simulink model "baseline_auto_parcel_loading_process"  (R2026a)
settings: Solver=VariableStepAuto  StopTime=500  MaxStep=0.05
libraries: sim3dlib x36
(part 3 of 5)

== matlab function baseline_auto_parcel_loading_process/Sim3DMappingFunction ==
  data: platform_z input; platform_x output; rotator_angle input; pusher_pos input; stopper_pos input; platform_fold_angle input; platform_y output; platform_z_3d output; platform_translation output; platform_rotation output; platform_scale output; rotator_x output; rotator_y output; rotator_z output; rotator_yaw output; rotator_translation output; rotator_rotation output; rotator_scale output; pusher_x output; pusher_y output; pusher_z output; pusher_translation output; pusher_rotation output; pusher_scale output; stopper1_translation output; stopper2_translation output; stopper3_translation output; stopper_rotation output; stopper_scale output; mission_phase input
function [platform_x, platform_y, platform_z_3d, platform_translation, platform_rotation, platform_scale, ...
    rotator_x, rotator_y, rotator_z, rotator_yaw, rotator_translation, rotator_rotation, rotator_scale, ...
    pusher_x, pusher_y, pusher_z, pusher_translation, pusher_rotation, pusher_scale, ...
    stopper1_translation, stopper2_translation, stopper3_translation, stopper_rotation, stopper_scale] = ...
    Sim3DMappingFunction(platform_z, rotator_angle, pusher_pos, stopper_pos, platform_fold_angle, mission_phase)
% Sim3DMappingFunction
% Simulink 제어 신호를 3D 객체 위치/회전 신호로 변환한다.
%
% 입력:
% platform_z          : 실제 플랫폼 높이
% rotator_angle       : 플랫폼 위 회전판 yaw 각도
% pusher_pos          : 푸셔 전진 위치
% stopper_pos         : 스토퍼 위치, 1=세움, 0=접힘
% platform_fold_angle : 플랫폼 접힘 각도, 0=펼침, pi/2=접힘
% mission_phase       : 0=상차, 1=하차 준비/하차, 2=미션 완료

% =========================
% 기준 위치
% =========================
platform_base_x = 0.0;
platform_base_y = -0.35;

rotator_offset_x = 0.0;
rotator_offset_y = 0.0;
rotator_offset_z = 0.02;

pusher_offset_y_home = -0.16;
pusher_offset_z = 0.055;

% =========================
% 층 높이
% =========================
z_floor1 = 0.00;
z_floor2 = 0.27;
z_floor3 = 0.54;

% =========================
% 플랫폼 위치
% =========================
platform_x = platform_base_x;
platform_y = platform_base_y;
platform_z_visual_offset = -0.02;
platform_z_3d = platform_z + platform_z_visual_offset;

platform_translation = [platform_x, platform_y, platform_z_3d];

% platform_fold_angle:
% 0      = 펼침
% pi/2   = 접힘
%
% 접히는 축이 이상하면 여기만 바꾸면 됨.
platform_rotation = [platform_fold_angle, 0, 0];

platform_scale = [1, 1, 1];

% 거의 펼쳐진 상태인지 판단
platform_deployed = 0;
if platform_fold_angle < 0.05
    platform_deployed = 1;
end

% =========================
% 회전판 위치/회전
% =========================
rotator_x = platform_x + rotator_offset_x;
rotator_y = platform_y + rotator_offset_y;
rotator_z = platform_z_3d + rotator_offset_z;
rotator_yaw = rotator_angle;

if platform_deployed > 0.5
    rotator_translation = [rotator_x, rotator_y, rotator_z];
    rotator_rotation    = [0, 0, rotator_yaw];
    rotator_scale       = [1, 1, 1];
else
    % 플랫폼이 접힌 상태에서는 회전판 숨김
    rotator_translation = [rotator_x, rotator_y, -10.0];
    rotator_rotation    = [0, 0, 0];
    rotator_scale       = [1, 1, 1];
end

% =========================
% 푸셔 위치
% =========================
pusher_x = platform_x;
pusher_y = platform_y + pusher_offset_y_home + pusher_pos;
pusher_z = platform_z_3d + pusher_offset_z;

if platform_deployed > 0.5
    pusher_translation = [pusher_x, pusher_y, pusher_z];
    pusher_rotation    = [0, 0, 0];
    pusher_scale       = [1, 1, 1];
else
    % 플랫폼이 접힌 상태에서는 푸셔 숨김
    pusher_translation = [pusher_x, pusher_y, -10.0];
    pusher_rotation    = [0, 0, 0];
    pusher_scale       = [1, 1, 1];
end

% =========================
% 층별 접이식 스토퍼 위치/회전
% =========================
stopper_base_x = -0.15;
stopper_base_y = platform_y + 0.30;

stopper_z_offset_on_belt = 0.05;

stopper1_x = stopper_base_x;
stopper1_y = stopper_base_y;
stopper1_z = z_floor1 + stopper_z_offset_on_belt;

stopper2_x = stopper_base_x;
stopper2_y = stopper_base_y;
stopper2_z = z_floor2 + stopper_z_offset_on_belt;

stopper3_x = stopper_base_x;
stopper3_y = stopper_base_y;
stopper3_z = z_floor3 + stopper_z_offset_on_belt;

if mission_phase == 0
    % 상차 중: 스토퍼 표시
    stopper1_translation = [stopper1_x, stopper1_y, stopper1_z];
    stopper2_translation = [stopper2_x, stopper2_y, stopper2_z];
    stopper3_translation = [stopper3_x, stopper3_y, stopper3_z];

    stopper_fold_angle = (pi/2) * (1 - stopper_pos);
    stopper_rotation = [0, stopper_fold_angle, 0];

    stopper_scale = [1, 1, 1];

else
    % 하차 준비/하차/완료 중: 스토퍼 숨김
    hide_z = -10.0;

    stopper1_translation = [stopper1_x, stopper1_y, hide_z];
    stopper2_translation = [stopper2_x, stopper2_y, hide_z];
    stopper3_translation = [stopper3_x, stopper3_y, hide_z];

    stopper_rotation = [0, pi/2, 0];
    stopper_scale = [1, 1, 1];
end

end

== matlab function baseline_auto_parcel_loading_process/Conveyor3DMappingFunction ==
  data: platform_y input; belt1_f1_T output; belt2_f1_T output; belt3_f1_T output; belt4_f1_T output; belt1_f2_T output; belt2_f2_T output; belt3_f2_T output; belt4_f2_T output; belt1_f3_T output; belt2_f3_T output; belt3_f3_T output; belt4_f3_T output; belt1_S output; belt2_S output; belt3_S output; belt4_S output; belt_R output
function [belt1_f1_T, belt2_f1_T, belt3_f1_T, belt4_f1_T, ...
          belt1_f2_T, belt2_f2_T, belt3_f2_T, belt4_f2_T, ...
          belt1_f3_T, belt2_f3_T, belt3_f3_T, belt4_f3_T, ...
          belt1_S, belt2_S, belt3_S, belt4_S, ...
          belt_R] = Conveyor3DMappingFunction_v3(platform_y)
% Conveyor3DMappingFunction_v3
% 3층 순환 컨베이어 4개 벨트의 3D 좌표 생성
%
% 1층에서 확정한 형상을 z 방향으로 복제한다.
%
% 진행 방향:
% Belt3: +x 방향
% Belt4: side_y 방향
% Belt1: -x 방향
% Belt2: Belt1 끝에서 Belt3 쪽으로 복귀
%
% 길이:
% Belt2, Belt4 = 1.11 m
% Belt1, Belt3 = 0.51 m
% 폭 = 0.25 m
%
% 중요:
% belt4_platform_extend = 0.25로 확정

% =========================
% 기본 치수
% =========================
belt_width = 0.25;      % 250 mm
belt_thick = 0.015;

L1 = 0.51;              % Belt1 length
L2 = 1.11;              % Belt2 기준 length
L3 = 0.51;              % Belt3 length
L4 = 1.11;              % Belt4 기준 length

% =========================
% 고정된 스토퍼/Belt3 기준
% =========================
stopper_x = -0.15;
stopper_y = platform_y + 0.30;
stopper_thick_x = 0.03;

% Belt3 끝점 A
A_x = stopper_x - stopper_thick_x/2;
A_y = stopper_y;

% =========================
% 방향 설정
% =========================
side_y = 1;
side_x = 1;

% =========================
% 층 높이
% =========================
z_floor1 = 0.00;
z_floor2 = 0.27;
z_floor3 = 0.54;

% 플랫폼/벨트 윗면 기준
% 각 층에서 벨트 윗면이 해당 층 z_floor와 같도록 설정
belt_center_z_f1 = z_floor1 - belt_thick/2;
belt_center_z_f2 = z_floor2 - belt_thick/2;
belt_center_z_f3 = z_floor3 - belt_thick/2;

% =========================================================
% Belt3: 기준 벨트, 위치 고정
% 진행 방향 +x, 오른쪽 끝이 A점
% =========================================================
belt3_right_x = A_x;
belt3_left_x  = belt3_right_x - L3;

belt3_center_x = (belt3_left_x + belt3_right_x) / 2;
belt3_center_y = A_y;

belt3_connect_edge_y = belt3_center_y + side_y * belt_width/2;

% =========================================================
% Belt4
% =========================================================
if side_x > 0
    belt4_left_x  = A_x;
    belt4_right_x = A_x + belt_width;
else
    belt4_left_x  = A_x - belt_width;
    belt4_right_x = A_x;
end

belt4_center_x = (belt4_left_x + belt4_right_x) / 2;

belt4_start_y_nominal = belt3_connect_edge_y;

% 확정값
belt4_platform_extend = 0.25;

belt4_start_y = belt4_start_y_nominal - side_y * belt4_platform_extend;
belt4_end_y   = belt4_start_y_nominal + side_y * L4;

belt4_center_y = (belt4_start_y + belt4_end_y) / 2;
L4_actual = abs(belt4_end_y - belt4_start_y);

if side_x > 0
    belt4_outer_x = belt4_right_x;
else
    belt4_outer_x = belt4_left_x;
end

belt4_end_edge_y = belt4_end_y;

% =========================================================
% Belt1
% =========================================================
belt1_right_x = belt4_outer_x;
belt1_left_x  = belt1_right_x - L1;

belt1_center_x = (belt1_left_x + belt1_right_x) / 2;

belt1_inner_edge_y = belt4_end_edge_y;
belt1_center_y = belt1_inner_edge_y + side_y * belt_width/2;

belt1_outer_edge_y = belt1_inner_edge_y + side_y * belt_width;

% =========================================================
% Belt2
% =========================================================
belt2_right_x = belt1_left_x;
belt2_left_x  = belt2_right_x - belt_width;
belt2_center_x = (belt2_left_x + belt2_right_x) / 2;

belt2_start_y = belt1_outer_edge_y;
belt2_end_y   = belt3_connect_edge_y;
belt2_center_y = (belt2_start_y + belt2_end_y) / 2;

L2_actual = abs(belt2_start_y - belt2_end_y);

% =========================
% 1층 Translation
% =========================
belt1_f1_T = [belt1_center_x, belt1_center_y, belt_center_z_f1];
belt2_f1_T = [belt2_center_x, belt2_center_y, belt_center_z_f1];
belt3_f1_T = [belt3_center_x, belt3_center_y, belt_center_z_f1];
belt4_f1_T = [belt4_center_x, belt4_center_y, belt_center_z_f1];

% =========================
% 2층 Translation
% =========================
belt1_f2_T = [belt1_center_x, belt1_center_y, belt_center_z_f2];
belt2_f2_T = [belt2_center_x, belt2_center_y, belt_center_z_f2];
belt3_f2_T = [belt3_center_x, belt3_center_y, belt_center_z_f2];
belt4_f2_T = [belt4_center_x, belt4_center_y, belt_center_z_f2];

% =========================
% 3층 Translation
% =========================
belt1_f3_T = [belt1_center_x, belt1_center_y, belt_center_z_f3];
belt2_f3_T = [belt2_center_x, belt2_center_y, belt_center_z_f3];
belt3_f3_T = [belt3_center_x, belt3_center_y, belt_center_z_f3];
belt4_f3_T = [belt4_center_x, belt4_center_y, belt_center_z_f3];

% =========================
% Scale
% 모든 층에서 동일하게 사용
% =========================
belt1_S = [L1, belt_width, belt_thick];
belt2_S = [belt_width, L2_actual, belt_thick];
belt3_S = [L3, belt_width, belt_thick];
belt4_S = [belt_width, L4_actual, belt_thick];

belt_R = [0, 0, 0];

== matlab function baseline_auto_parcel_loading_process/Package3DMappingFunction_F2 ==
  data: floor2_visual_id input size=[6 1]; floor2_visible input size=[50 1]; floor2_color_flag input size=[50 1]; platform_y input size=[1 1]; floor2_visual_count input size=[1 1]; target_unload_id input size=[1 1]; highlight_enable input size=[1 1]; pkg1_T output; pkg2_T output; pkg3_T output; pkg4_T output; pkg5_T output; pkg1_R output; pkg2_R output; pkg3_R output; pkg4_R output; pkg5_R output; pkg1_S output; pkg2_S output; pkg3_S output; pkg4_S output; pkg5_S output; pkg6_T output; pkg6_R output; pkg6_S output; pkg1_Color output; pkg2_Color output; pkg3_Color output; pkg4_Color output; pkg5_Color output; pkg6_Color output; target_package_on_belt4 input size=[1 1]; package_on_platform_from_floor input size=[1 1]; platform_z input size=[1 1]; current_unload_id input size=[1 1]; floor2_visual_path input size=[6 1]; target_list input size=[20 1]; target_count input size=[1 1]; belt4_reverse_progress input size=[1 1]; belt4_reverse_phase input size=[1 1]
function [pkg1_T, pkg2_T, pkg3_T, pkg4_T, pkg5_T, ...
          pkg1_R, pkg2_R, pkg3_R, pkg4_R, pkg5_R, ...
          pkg1_S, pkg2_S, pkg3_S, pkg4_S, pkg5_S, ...
          pkg6_T, pkg6_R, pkg6_S, ...
          pkg1_Color, pkg2_Color, pkg3_Color, pkg4_Color, pkg5_Color, pkg6_Color] = ...
          Package3DMappingFunction_F2(floor2_visual_id, floor2_visible, floor2_color_flag, platform_y, floor2_visual_count, ...
                                      target_unload_id, highlight_enable, target_package_on_belt4, ...
                                      package_on_platform_from_floor, platform_z, current_unload_id, floor2_visual_path, ...
                                      target_list, target_count, belt4_reverse_progress, belt4_reverse_phase)
% Package3DMappingFunction_F2
% 2층 정적/연속 이동 박스 표시 함수
%
% 중요:
% - 이제 F2는 FloorStorageUpdate/floor2_queue 또는 PackageSlotVisualizer/floor2_slot_id를 직접 쓰지 않는다.
% - Floor2VisualStateFunction이 저장한 floor2_visual_id, floor2_visual_path를 기준으로 표시한다.
% - visual_shift는 이 함수에 직접 들어오지 않는다.
%
% 입력:
% floor2_visual_id               [6x1]
% floor2_visible                 [50x1]  % 기존 포트 유지용
% floor2_color_flag              [50x1]  % 기존 포트 유지용
% platform_y                     [1x1]
% floor2_visual_count            [1x1]
% target_unload_id               [1x1]  % 2층 하차공간 준비 대상
% highlight_enable               [1x1]
% target_package_on_belt4        [1x1]
% package_on_platform_from_floor [1x1]
% platform_z                     [1x1]
% current_unload_id              [1x1]  % 현재 실제 하차 대상
% floor2_visual_path             [6x1]

% =========================
% 박스 크기
% =========================
pkg_short = 0.12;
pkg_long  = 0.16;
pkg_h     = 0.08;

pkg_scale = [pkg_short, pkg_long, pkg_h];

% =========================
% 색상 설정
% =========================
normal_color = [0.75, 0.45, 0.20];
target_color = [1.0, 1.0, 0.0];

% =========================
% 2층 높이
% =========================
z_floor2 = 0.27;
pkg_center_z = z_floor2 + pkg_h / 2;

hide_z = -10.0;

% =========================
% 컨베이어 기준값
% =========================
belt_width = 0.25;

L1 = 0.51;
L3 = 0.51;
L4 = 1.11;

stopper_x = -0.15;
stopper_y = platform_y + 0.30;
stopper_thick_x = 0.03;

A_x = stopper_x - stopper_thick_x / 2;
A_y = stopper_y;

side_y = 1;
side_x = 1;

% =========================
% Belt3 geometry
% =========================
belt3_right_x = A_x;
belt3_center_y = A_y;
belt3_connect_edge_y = belt3_center_y + side_y * belt_width / 2;

% =========================
% Belt4 geometry
% =========================
if side_x > 0
    belt4_left_x  = A_x;
    belt4_right_x = A_x + belt_width;
else
    belt4_left_x  = A_x - belt_width;
    belt4_right_x = A_x;
end

belt4_center_x = (belt4_left_x + belt4_right_x) / 2;

belt4_start_y_nominal = belt3_connect_edge_y;
belt4_platform_extend = 0.25;

belt4_start_y = belt4_start_y_nominal - side_y * belt4_platform_extend;
belt4_end_y = belt4_start_y_nominal + side_y * L4;

if side_x > 0
    belt4_outer_x = belt4_right_x;
else
    belt4_outer_x = belt4_left_x;
end

% =========================
% 하차공간 좌표
% =========================
handoff_x = belt4_center_x;
handoff_y = belt4_start_y + side_y * (pkg_short / 2 + 0.02);
handoff_z = pkg_center_z;
handoff_yaw = pi / 2;

% Belt4 앞쪽 최대 위치 제한
belt4_max_y = belt4_end_y - side_y * (pkg_short / 2 + 0.02);

% =========================
% 플랫폼 위 회수 박스 좌표
% =========================
platform_pkg_x = 0.0;
platform_pkg_y = platform_y ;
platform_pkg_z = platform_z + pkg_h / 2;
platform_pkg_yaw = pi / 2;

% =========================
% Belt1 geometry
% =========================
belt1_right_x = belt4_outer_x;
belt1_left_x  = belt1_right_x - L1;

belt1_inner_edge_y = belt4_end_y;
belt1_outer_edge_y = belt1_inner_edge_y + side_y * belt_width;

% =========================
% Belt2 geometry
% =========================
belt2_right_x = belt1_left_x;
belt2_left_x  = belt2_right_x - belt_width;
belt2_center_x = (belt2_left_x + belt2_right_x) / 2;

belt2_end_y = belt3_connect_edge_y;

% =========================
% 슬롯 배치 파라미터
% =========================
max_on_belt3 = 4;

pkg_visual_gap = 0.005;
slot_pitch = pkg_short + pkg_visual_gap;

stopper_center_gap = pkg_short / 2;
belt2_entry_gap = 0.04;

% =========================
% 기존 입력 포트 사용 처리
% =========================
% floor2_visible, floor2_color_flag는 기존 모델 연결을 유지하기 위한 입력이다.
% 현재 F2는 floor2_visual_id/path 기준으로 동작한다.
dummy_keep = floor2_visible(1) + floor2_color_flag(1);
dummy_keep = dummy_keep + 0;

% =========================
% 표시 여부
% =========================
visible1 = (floor2_visual_id(1) > 0);
visible2 = (floor2_visual_id(2) > 0);
visible3 = (floor2_visual_id(3) > 0);
visible4 = (floor2_visual_id(4) > 0);
visible5 = (floor2_visual_id(5) > 0);
visible6 = (floor2_visual_id(6) > 0);
% =========================
% 각 박스 생성
% =========================
[pkg1_T, pkg1_R, pkg1_S, pkg1_Color] = makePkg(floor2_visual_id(1), floor2_visual_path(1), visible1, ...
    belt3_right_x, belt3_center_y, belt2_center_x, belt2_end_y, ...
    belt4_center_x, belt4_max_y, ...
    slot_pitch, stopper_center_gap, belt2_entry_gap, max_on_belt3, ...
    pkg_center_z, hide_z, pkg_scale, side_y, ...
    target_unload_id, highlight_enable, target_package_on_belt4, ...
    handoff_x, handoff_y, handoff_z, handoff_yaw, ...
    package_on_platform_from_floor, platform_pkg_x, platform_pkg_y, platform_pkg_z, platform_pkg_yaw, ...
    current_unload_id, normal_color, target_color, target_list, target_count, belt4_reverse_progress, belt4_reverse_phase);

[pkg2_T, pkg2_R, pkg2_S, pkg2_Color] = makePkg(floor2_visual_id(2), floor2_visual_path(2), visible2, ...
    belt3_right_x, belt3_center_y, belt2_center_x, belt2_end_y, ...
    belt4_center_x, belt4_max_y, ...
    slot_pitch, stopper_center_gap, belt2_entry_gap, max_on_belt3, ...
    pkg_center_z, hide_z, pkg_scale, side_y, ...
    target_unload_id, highlight_enable, target_package_on_belt4, ...
    handoff_x, handoff_y, handoff_z, handoff_yaw, ...
    package_on_platform_from_floor, platform_pkg_x, platform_pkg_y, platform_pkg_z, platform_pkg_yaw, ...
    current_unload_id, normal_color, target_color, target_list, target_count, belt4_reverse_progress, belt4_reverse_phase);

[pkg3_T, pkg3_R, pkg3_S, pkg3_Color] = makePkg(floor2_visual_id(3), floor2_visual_path(3), visible3, ...
    belt3_right_x, belt3_center_y, belt2_center_x, belt2_end_y, ...
    belt4_center_x, belt4_max_y, ...
    slot_pitch, stopper_center_gap, belt2_entry_gap, max_on_belt3, ...
    pkg_center_z, hide_z, pkg_scale, side_y, ...
    target_unload_id, highlight_enable, target_package_on_belt4, ...
    handoff_x, handoff_y, handoff_z, handoff_yaw, ...
    package_on_platform_from_floor, platform_pkg_x, platform_pkg_y, platform_pkg_z, platform_pkg_yaw, ...
    current_unload_id, normal_color, target_color, target_list, target_count, belt4_reverse_progress, belt4_reverse_phase);

[pkg4_T, pkg4_R, pkg4_S, pkg4_Color] = makePkg(floor2_visual_id(4), floor2_visual_path(4), visible4, ...
    belt3_right_x, belt3_center_y, belt2_center_x, belt2_end_y, ...
    belt4_center_x, belt4_max_y, ...
    slot_pitch, stopper_center_gap, belt2_entry_gap, max_on_belt3, ...
    pkg_center_z, hide_z, pkg_scale, side_y, ...
    target_unload_id, highlight_enable, target_package_on_belt4, ...
    handoff_x, handoff_y, handoff_z, handoff_yaw, ...
    package_on_platform_from_floor, platform_pkg_x, platform_pkg_y, platform_pkg_z, platform_pkg_yaw, ...
    current_unload_id, normal_color, target_color, target_list, target_count, belt4_reverse_progress, belt4_reverse_phase);

[pkg5_T, pkg5_R, pkg5_S, pkg5_Color] = makePkg(floor2_visual_id(5), floor2_visual_path(5), visible5, ...
    belt3_right_x, belt3_center_y, belt2_center_x, belt2_end_y, ...
    belt4_center_x, belt4_max_y, ...
    slot_pitch, stopper_center_gap, belt2_entry_gap, max_on_belt3, ...
    pkg_center_z, hide_z, pkg_scale, side_y, ...
    target_unload_id, highlight_enable, target_package_on_belt4, ...
    handoff_x, handoff_y, handoff_z, handoff_yaw, ...
    package_on_platform_from_floor, platform_pkg_x, platform_pkg_y, platform_pkg_z, platform_pkg_yaw, ...
    current_unload_id, normal_color, target_color, target_list, target_count, belt4_reverse_progress, belt4_reverse_phase);

[pkg6_T, pkg6_R, pkg6_S, pkg6_Color] = makePkg(floor2_visual_id(6), floor2_visual_path(6), visible6, ...
    belt3_right_x, belt3_center_y, belt2_center_x, belt2_end_y, ...
    belt4_center_x, belt4_max_y, ...
    slot_pitch, stopper_center_gap, belt2_entry_gap, max_on_belt3, ...
    pkg_center_z, hide_z, pkg_scale, side_y, ...
    target_unload_id, highlight_enable, target_package_on_belt4, ...
    handoff_x, handoff_y, handoff_z, handoff_yaw, ...
    package_on_platform_from_floor, platform_pkg_x, platform_pkg_y, platform_pkg_z, platform_pkg_yaw, ...
    current_unload_id, normal_color, target_color, target_list, target_count, belt4_reverse_progress, belt4_reverse_phase);

end


function [T, R, S, C] = makePkg(package_id, visual_path, visible, ...
                                 belt3_right_x, belt3_y, ...
                                 belt2_x, belt2_entry_y, ...
                                 belt4_center_x, belt4_max_y, ...
                                 slot_pitch, stopper_center_gap, belt2_entry_gap, ...
                                 max_on_belt3, pkg_center_z, hide_z, pkg_scale, side_y, ...
                                 target_unload_id, highlight_enable, target_package_on_belt4, ...
                                 handoff_x, handoff_y, handoff_z, handoff_yaw, ...
                                 package_on_platform_from_floor, platform_pkg_x, platform_pkg_y, platform_pkg_z, platform_pkg_yaw, ...
                                 current_unload_id, normal_color, target_color, target_list, target_count, belt4_reverse_progress, belt4_reverse_phase);

C = normal_color;

% 상차 완료 후에만 target_list 안의 하차 대상 전체를 노란색으로 표시
if highlight_enable > 0.5
    if isUnloadTarget(package_id, target_list, target_count) > 0.5
        C = target_color;
    end
end

% 플랫폼 위에 올라간 현재 하차 대상도 노란색 유지
if package_on_platform_from_floor > 0.5 && package_id == current_unload_id && package_id > 0
    C = target_color;
end

if visible > 0.5 && package_id > 0

    % 1순위: Belt4 역회전으로 현재 하차대상 박스를 플랫폼까지 밀기
    if belt4_reverse_phase == 1 && belt4_reverse_progress > 0 && package_id == current_unload_id && package_id > 0

        p = belt4_reverse_progress;

        if p < 0
            p = 0;
        end

        if p > 1
            p = 1;
        end

        push_to_x = platform_pkg_x;

        % 방향이 반대면 -를 +로 바꿔야 함
        push_to_y = handoff_y - side_y * 0.40;

        push_to_z = platform_pkg_z;

        x = handoff_x + p * (push_to_x - handoff_x);
        y = handoff_y + p * (push_to_y - handoff_y);
        z = handoff_z + p * (push_to_z - handoff_z);

        T = [x, y, z];
        R = [0, 0, platform_pkg_yaw];
        S = pkg_scale;
        C = target_color;
        return;
    end

    % 2순위: 플랫폼 위에 완전히 올라간 상태
    if package_on_platform_from_floor > 0.5 && package_id == current_unload_id && package_id > 0
        T = [platform_pkg_x, platform_pkg_y, platform_pkg_z];
        R = [0, 0, platform_pkg_yaw];
        S = pkg_scale;
        C = target_color;
        return;
    end

    % 3순위: visual_path 위치
    [x, y, yaw] = getContinuousPose(visual_path, ...
        belt3_right_x, belt3_y, ...
        belt2_x, belt2_entry_y, ...
        belt4_center_x, belt4_max_y, ...
        slot_pitch, stopper_center_gap, belt2_entry_gap, ...
        max_on_belt3, side_y, ...
        handoff_x, handoff_y, handoff_yaw);

    T = [x, y, pkg_center_z];
    R = [0, 0, yaw];
    S = pkg_scale;

else
    T = [0, 0, hide_z];
    R = [0, 0, 0];
    S = pkg_scale;
end

end


function [x, y, yaw] = getContinuousPose(path_pos, ...
                                         belt3_right_x, belt3_y, ...
                                         belt2_x, belt2_entry_y, ...
                                         belt4_center_x, belt4_max_y, ...
                                         slot_pitch, stopper_center_gap, belt2_entry_gap, ...
                                         max_on_belt3, side_y, ...
                                         handoff_x, handoff_y, handoff_yaw)
% getContinuousPose
%
% path_pos 기준:
% path_pos = 4 : 기존 slot4 위치
% path_pos = 3 : 기존 slot3 위치
% path_pos = 2 : 기존 slot2 위치
% path_pos = 1 : 기존 slot1 위치
% path_pos = 0 : 하차공간
% path_pos < 0 : 하차공간보다 앞쪽 Belt4 위

upper_idx = ceil(path_pos);
lower_idx = floor(path_pos);

if upper_idx == lower_idx
    [x, y, yaw] = getIntegerPose(upper_idx, ...
        belt3_right_x, belt3_y, ...
        belt2_x, belt2_entry_y, ...
        belt4_center_x, belt4_max_y, ...
        slot_pitch, stopper_center_gap, belt2_entry_gap, ...
        max_on_belt3, side_y, ...
        handoff_x, handoff_y, handoff_yaw);
else
    alpha = upper_idx - path_pos;

    if alpha < 0
        alpha = 0;
    end

    if alpha > 1
        alpha = 1;
    end

    [x_upper, y_upper, yaw_upper] = getIntegerPose(upper_idx, ...
        belt3_right_x, belt3_y, ...
        belt2_x, belt2_entry_y, ...
        belt4_center_x, belt4_max_y, ...
        slot_pitch, stopper_center_gap, belt2_entry_gap, ...
        max_on_belt3, side_y, ...
        handoff_x, handoff_y, handoff_yaw);

    [x_lower, y_lower, yaw_lower] = getIntegerPose(lower_idx, ...
        belt3_right_x, belt3_y, ...
        belt2_x, belt2_entry_y, ...
        belt4_center_x, belt4_max_y, ...
        slot_pitch, stopper_center_gap, belt2_entry_gap, ...
        max_on_belt3, side_y, ...
        handoff_x, handoff_y, handoff_yaw);

    x = x_upper + alpha * (x_lower - x_upper);
    y = y_upper + alpha * (y_lower - y_upper);

    if alpha < 0.5
        yaw = yaw_upper;
    else
        yaw = yaw_lower;
    end
end

end


function [x, y, yaw] = getIntegerPose(idx, ...
                                      belt3_right_x, belt3_y, ...
                                      belt2_x, belt2_entry_y, ...
                                      belt4_center_x, belt4_max_y, ...
                                      slot_pitch, stopper_center_gap, belt2_entry_gap, ...
                                      max_on_belt3, side_y, ...
                                      handoff_x, handoff_y, handoff_yaw)
% getIntegerPose
%
% idx >= 1:
%   기존 Belt3/Belt2 슬롯 위치
%
% idx == 0:
%   하차공간
%
% idx < 0:
%   하차공간보다 더 앞쪽의 Belt4 위치

if idx <= 0

    x = belt4_center_x;
    y = handoff_y + side_y * (-idx) * slot_pitch;

    if side_y > 0
        if y > belt4_max_y
            y = belt4_max_y;
        end
    else
        if y < belt4_max_y
            y = belt4_max_y;
        end
    end

    yaw = handoff_yaw;

elseif idx <= max_on_belt3

    d = stopper_center_gap + slot_pitch * (idx - 1);

    x = belt3_right_x - d;
    y = belt3_y;

    yaw = 0;

else

    k = idx - max_on_belt3;

    x = belt2_x;
    y = belt2_entry_y + side_y * (belt2_entry_gap + slot_pitch * (k - 1));

    yaw = pi / 2;

end

end

function flag = isUnloadTarget(package_id, target_list, target_count)
% isUnloadTarget
%
% target_list 안에 package_id가 있으면 1, 없으면 0 반환
%
% target_list  [20x1]
% target_count [1x1]

flag = 0;

if package_id <= 0
    return;
end

n = target_count;

if n < 0
    n = 0;
end

if n > 20
    n = 20;
end

for i = 1:20
    if i <= n
        if target_list(i) == package_id
            flag = 1;
        end
    end
end

end

== matlab function baseline_auto_parcel_loading_process/MovingPackage3DMappingFunction ==
  data: mission_phase input; moving_pkg_T output; state_id input; platform_z_3d input; rotator_yaw input; pusher_pos input; platform_y input; moving_pkg_R output; moving_pkg_S output; box_yaw input; load_done input; rotation_done input; visual_count input; moving_arrive_done output; moving_arrive_floor output; target_floor input
function [moving_pkg_T, moving_pkg_R, moving_pkg_S, moving_arrive_done, moving_arrive_floor] ...
    = MovingPackage3DMappingFunction( ...
    mission_phase, state_id, platform_z_3d, rotator_yaw, pusher_pos, platform_y, box_yaw, load_done, rotation_done, visual_count, target_floor)% MovingPackage3DMappingFunction
% 동적 택배 1개를 플랫폼 → 푸셔 → Belt4 → Belt1 → Belt2 → Belt3/스토퍼 앞 위치까지 이동시킨다.
%
% 주의:
% - spawn_pkg 없이 동작하는 버전
% - load_done으로 박스를 숨기지 않음
% - moving_arrive_done이 1이 되는 순간 VisualArrivalCounterFunction이 visual_count를 증가시킴
% - Package3DMappingFunction은 visual_count 이하의 정적 박스만 표시함
%
% 출력:
% moving_pkg_T = [x y z]
% moving_pkg_R = [roll pitch yaw]
% moving_pkg_S = [sx sy sz]
% moving_arrive_done = 도착 순간 1펄스

% =========================
% Persistent 상태
% =========================
persistent active
persistent latched_yaw
persistent yaw_locked
persistent prev_rotation_done
persistent pushed_distance_max
persistent path_started
persistent path_s
persistent current_yaw_rad
persistent latched_pkg_z
persistent waiting_for_next_cycle
persistent visual_count_at_start
persistent target_slot_latched
persistent box_detached
persistent detach_z
persistent target_floor_latched
persistent smooth_yaw_initialized

if isempty(smooth_yaw_initialized)
    smooth_yaw_initialized = false;
end

if isempty(target_floor_latched)
    target_floor_latched = 2;
end

if isempty(box_detached)
    box_detached = false;
end

if isempty(detach_z)
    detach_z = 0;
end

if isempty(active)
    active = false;
end

if isempty(latched_yaw)
    latched_yaw = 0;
end

if isempty(yaw_locked)
    yaw_locked = false;
end

if isempty(prev_rotation_done)
    prev_rotation_done = 0;
end

if isempty(pushed_distance_max)
    pushed_distance_max = 0;
end

if isempty(path_started)
    path_started = false;
end

if isempty(path_s)
    path_s = 0;
end

if isempty(current_yaw_rad)
    current_yaw_rad = pi/2;
end

if isempty(latched_pkg_z)
    latched_pkg_z = 0;
end

if isempty(waiting_for_next_cycle)
    waiting_for_next_cycle = false;
end

if isempty(visual_count_at_start)
    visual_count_at_start = 0;
end

if isempty(target_slot_latched)
    target_slot_latched = 1;
end

% 기본 출력
moving_arrive_done = 0;
moving_arrive_floor = 0;
rotation_done_rising = (rotation_done > 0.5) && (prev_rotation_done <= 0.5);
debug_active = 0;
debug_waiting = 0;
debug_start_allowed = 0;
debug_target_slot = target_slot_latched;
debug_visual_count = visual_count;
debug_mission_phase = mission_phase;

% =========================
% 박스 크기
% =========================
pkg_short = 0.12;
pkg_long  = 0.16;
pkg_h     = 0.08;

moving_pkg_S = [pkg_short, pkg_long, pkg_h];

% =========================
% 플랫폼 기준 위치
% =========================
platform_x = 0.0;
pkg_home_x = platform_x;
pkg_home_y = platform_y;

platform_thickness = 0.04;
pkg_center_z_now = platform_z_3d + platform_thickness/2 + pkg_h/2;

hide_z = -10.0;

% =========================
% 이벤트 감지
% =========================
rotation_done_rising = (rotation_done > 0.5) && (prev_rotation_done <= 0.5);

% =========================
% 플랫폼 위 정렬 목표 yaw
% yaw = pi/2이면 박스 짧은 변 0.12m가 +y 방향, 즉 푸셔 진행방향을 향함
% =========================
platform_aligned_yaw_rad = pi/2;

% =========================
% 다음 사이클 대기 해제
% =========================
% MovingPackage가 도착해서 visual_count가 증가한 뒤,
% 푸셔/회전/등록 신호가 초기화되면 다음 박스 생성 허용
if waiting_for_next_cycle
    same_floor_count_increased = (target_floor == target_floor_latched) && ...
                                 (visual_count > visual_count_at_start);

    floor_changed = (target_floor ~= target_floor_latched);

    if (same_floor_count_increased || floor_changed) && ...
       (pusher_pos < 0.005) && ...
       (rotation_done < 0.5) && ...
       (load_done < 0.5)
        waiting_for_next_cycle = false;
    end
end

% =========================
% 새 박스 시작 조건
% =========================
% spawn_pkg가 없으므로 현재는 state와 초기 조건으로 시작을 추정한다.
% 추후 spawn_pkg를 만들면 이 부분을 spawn rising edge로 바꾸는 것이 가장 안정적이다.
start_allowed = (mission_phase == 0) && ...
                (active == false) && ...
                (waiting_for_next_cycle == false) && ...
                (pusher_pos < 0.005) && ...
                (rotation_done < 0.5) && ...
                (load_done < 0.5) && ...
                (state_id < 7);
if start_allowed
    active = true;
    latched_yaw = box_yaw;
    yaw_locked = false;
    pushed_distance_max = 0;
    path_started = false;
    path_s = 0;
    target_floor_latched = target_floor;

    box_detached = false;
    detach_z = pkg_center_z_now;

    current_yaw_rad = platform_aligned_yaw_rad + latched_yaw * pi / 180;
    smooth_yaw_initialized = true;
    latched_pkg_z = pkg_center_z_now;

    visual_count_at_start = visual_count;

    target_slot_latched = visual_count + 1;
    if target_slot_latched < 1
        target_slot_latched = 1;
    end
    if target_slot_latched > 6
        target_slot_latched = 6;
    end
end

% =========================
% 회전 완료 시 yaw 고정
% =========================
if active && rotation_done_rising
    yaw_locked = true;
end

% =========================
% 푸셔 최대 이동거리 저장
% =========================
if active
    if pusher_pos > pushed_distance_max
        pushed_distance_max = pusher_pos;
    end
end

% =========================
% 푸셔 완료 후 경로 이동 시작
% =========================
pusher_finished = pushed_distance_max >= 0.22;

if active && pusher_finished && box_detached == false
    box_detached = true;

    % 이 순간부터 박스는 플랫폼과 별개로 움직인다.
    % 따라서 현재 높이를 고정 저장한다.
    detach_z = pkg_center_z_now;
    latched_pkg_z = pkg_center_z_now;
end

if active && pusher_finished && path_started == false
    path_started = true;
    path_s = 0;

    yaw_locked = true;
    current_yaw_rad = platform_aligned_yaw_rad;
end

% =========================
% 경로 파라미터
% =========================
[path_total_length, seg1_end, seg2_end, seg3_end] = getPathLengths(platform_y, target_slot_latched);

% 이동 속도
path_speed_per_step = 0.012;

if active && path_started
    if path_s < path_total_length
        path_s = path_s + path_speed_per_step;
    end

    if path_s > path_total_length
        path_s = path_total_length;
    end
end

% =========================
% 하차/완료 phase에서는 강제 숨김
% =========================
%if mission_phase > 0
%    active = false;
%    yaw_locked = false;
%    pushed_distance_max = 0;
%    path_started = false;
%    path_s = 0;
%    waiting_for_next_cycle = true;
%    box_detached = false;
%    detach_z = 0;
%end

% =========================
% 출력 계산
% =========================
if active

    if path_started
        [x, y, target_yaw_rad] = getPathPose(path_s, platform_y, target_slot_latched, seg1_end, seg2_end, seg3_end);

        % 우선 빙글빙글 도는 문제 방지를 위해 yaw는 목표값으로 직접 지정한다.
        % 안정화 후 부드러운 회전을 다시 추가하면 된다.
        current_yaw_rad = target_yaw_rad;

        z = latched_pkg_z;

        moving_pkg_T = [x, y, z];
        moving_pkg_R = [0, 0, current_yaw_rad];

        if path_s >= path_total_length
            moving_arrive_done = 1;
            moving_arrive_floor = target_floor_latched;

            active = false;
            yaw_locked = false;
            pushed_distance_max = 0;
            path_started = false;
            path_s = 0;
            box_detached = false;
            detach_z = 0;

            waiting_for_next_cycle = true;
        end

    else
        % 플랫폼 위, 회전판 위, 푸셔 이동 구간
        push_visual_gain = 1.0;
        push_y = push_visual_gain * pushed_distance_max;

        x = pkg_home_x;
        y = pkg_home_y + push_y;
        if box_detached
            z = detach_z;
        else
            z = pkg_center_z_now;
        end

        moving_pkg_T = [x, y, z];

        % =========================
        % 플랫폼 위 박스 yaw 부드러운 목표각 추종
        % =========================
        % 중요:
        % - rotator_yaw를 직접 따라가면 목표각을 지나쳤다가 보정되는 현상이 생긴다.
        % - 시각화용 박스 yaw는 항상 최종 최소길이 목표각(platform_aligned_yaw_rad)만 바라보게 한다.
        % - 현재 yaw에서 목표 yaw까지 한 step씩 접근하므로 절대 목표각을 넘어가지 않는다.

        Ts_yaw = 0.05;
        yaw_speed = 1.2;     % rad/s, 더 빠르게 원하면 1.5~2.0
        yaw_step = yaw_speed * Ts_yaw;

        desired_yaw_rad = platform_aligned_yaw_rad;

        yaw_err = wrapToPiLocal(desired_yaw_rad - current_yaw_rad);

        if abs(yaw_err) <= yaw_step
            current_yaw_rad = desired_yaw_rad;
        else
            if yaw_err > 0
                current_yaw_rad = current_yaw_rad + yaw_step;
            else
                current_yaw_rad = current_yaw_rad - yaw_step;
            end
        end

        moving_pkg_R = [0, 0, current_yaw_rad];
    end

else
    moving_pkg_T = [0, 0, hide_z];
    moving_pkg_R = [0, 0, 0];
end


% =========================
% 이전값 저장
% =========================
prev_rotation_done = rotation_done;

end


function [path_total_length, seg1_end, seg2_end, seg3_end] = getPathLengths(platform_y_local, target_slot)
% 경로 길이 계산

belt_width = 0.25;
pkg_short = 0.12;
pkg_visual_gap = 0.005;
slot_pitch = pkg_short + pkg_visual_gap;

L1 = 0.51;
L3 = 0.51;
L4 = 1.11;

max_on_belt3 = 4;

stopper_x = -0.15;
stopper_y = platform_y_local + 0.30;
stopper_thick_x = 0.03;

A_x = stopper_x - stopper_thick_x/2;
A_y = stopper_y;

side_y = 1;
side_x = 1;

% Belt3
belt3_center_y = A_y;
belt3_connect_edge_y = belt3_center_y + side_y * belt_width/2;

% Belt4
if side_x > 0
    belt4_left_x  = A_x;
    belt4_right_x = A_x + belt_width;
else
    belt4_left_x  = A_x - belt_width;
    belt4_right_x = A_x;
end

belt4_start_y_nominal = belt3_connect_edge_y;
belt4_platform_extend = 0.25;

belt4_start_y = belt4_start_y_nominal - side_y * belt4_platform_extend;
belt4_end_y   = belt4_start_y_nominal + side_y * L4;

seg_belt4 = abs(belt4_end_y - belt4_start_y);

% Belt1
if side_x > 0
    belt4_outer_x = belt4_right_x;
else
    belt4_outer_x = belt4_left_x;
end

belt1_right_x = belt4_outer_x;
belt1_left_x  = belt1_right_x - L1;
seg_belt1 = abs(belt1_right_x - belt1_left_x);

% Belt2
belt1_inner_edge_y = belt4_end_y;
belt1_outer_edge_y = belt1_inner_edge_y + side_y * belt_width;

belt2_start_y = belt1_outer_edge_y;
belt2_end_y   = belt3_connect_edge_y;
seg_belt2_full = abs(belt2_start_y - belt2_end_y);

if target_slot <= max_on_belt3
    % 목표가 Belt3 위에 있음
    stopper_center_gap = pkg_short / 2;
    target_gap = stopper_center_gap + slot_pitch * (target_slot - 1);

    seg_belt3 = L3 - target_gap;

    if seg_belt3 < 0
        seg_belt3 = 0;
    end

    seg1_end = seg_belt4;
    seg2_end = seg_belt4 + seg_belt1;
    seg3_end = seg_belt4 + seg_belt1 + seg_belt2_full;
    path_total_length = seg_belt4 + seg_belt1 + seg_belt2_full + seg_belt3;

else
    % 목표가 Belt2 위에 있음
    % Belt4와 Belt1을 지난 뒤,
    % Belt2 시작점에서 목표 위치까지 실제 거리만큼 이동해야 한다.
    k = target_slot - max_on_belt3;

    belt2_entry_gap = 0.04;

    % Package3DMappingFunction의 정적 박스 위치와 동일한 목표 y
    % 6번째 박스가 5번째 박스 영역을 침범해 보이는 것을 막기 위한 동적 경로 보정
    % k = 1 : 5번째 박스
    % k = 2 : 6번째 박스
    moving_stop_margin = 0.01;

    target_y_on_belt2 = belt2_end_y + side_y * (belt2_entry_gap + slot_pitch * (k - 1) + moving_stop_margin);

    % 기존 오류:
    % seg_belt2_partial = belt2_entry_gap;
    % 이렇게 하면 0.04m만 이동해서 순간이동처럼 보임.
    %
    % 수정:
    % Belt2 시작점에서 target_y_on_belt2까지의 실제 거리 사용
    seg_belt2_partial = abs(belt2_start_y - target_y_on_belt2);

    seg1_end = seg_belt4;
    seg2_end = seg_belt4 + seg_belt1;
    seg3_end = seg2_end + seg_belt2_partial;
    path_total_length = seg_belt4 + seg_belt1 + seg_belt2_partial;
end

end


function [x, y, yaw_rad] = getPathPose(s, platform_y_local, target_slot, seg1_end, seg2_end, seg3_end)
% 경로상 위치와 yaw 계산

belt_width = 0.25;
pkg_short = 0.12;
pkg_visual_gap = 0.005;
slot_pitch = pkg_short + pkg_visual_gap;

L1 = 0.51;
L3 = 0.51;
L4 = 1.11;

max_on_belt3 = 4;

stopper_x = -0.15;
stopper_y = platform_y_local + 0.30;
stopper_thick_x = 0.03;

A_x = stopper_x - stopper_thick_x/2;
A_y = stopper_y;

side_y = 1;
side_x = 1;

% Belt3
belt3_right_x = A_x;
belt3_left_x  = belt3_right_x - L3;
belt3_center_y = A_y;
belt3_connect_edge_y = belt3_center_y + side_y * belt_width/2;

% Belt4
if side_x > 0
    belt4_left_x  = A_x;
    belt4_right_x = A_x + belt_width;
else
    belt4_left_x  = A_x - belt_width;
    belt4_right_x = A_x;
end

belt4_center_x = (belt4_left_x + belt4_right_x)/2;

belt4_start_y_nominal = belt3_connect_edge_y;
belt4_platform_extend = 0.25;

belt4_start_y = belt4_start_y_nominal - side_y * belt4_platform_extend;
belt4_end_y   = belt4_start_y_nominal + side_y * L4;

if side_x > 0
    belt4_outer_x = belt4_right_x;
else
    belt4_outer_x = belt4_left_x;
end

% Belt1
belt1_right_x = belt4_outer_x;
belt1_left_x  = belt1_right_x - L1;

belt1_inner_edge_y = belt4_end_y;
belt1_center_y = belt1_inner_edge_y + side_y * belt_width/2;
belt1_outer_edge_y = belt1_inner_edge_y + side_y * belt_width;

% Belt2
belt2_right_x = belt1_left_x;
belt2_left_x  = belt2_right_x - belt_width;
belt2_center_x = (belt2_left_x + belt2_right_x)/2;

belt2_start_y = belt1_outer_edge_y;
belt2_end_y   = belt3_connect_edge_y;

% target 위치
if target_slot <= max_on_belt3
    stopper_center_gap = pkg_short / 2;
    target_gap = stopper_center_gap + slot_pitch * (target_slot - 1);

    target_x = belt3_right_x - target_gap;
    target_y = belt3_center_y;
else
    k = target_slot - max_on_belt3;
    belt2_entry_gap = 0.04;

    % 동적 박스가 정적 박스 쪽을 살짝 침범해 보이는 것을 막기 위한 시각 보정
    % 값이 너무 크면 6번 박스가 뒤에 너무 떨어져 보이므로 0.01부터 시작
    % 6번째 박스가 5번째 박스 영역을 침범해 보이는 것을 막기 위한 동적 경로 보정
    % k = 1 : 5번째 박스
    % k = 2 : 6번째 박스
    moving_stop_margin = 0.01;

    target_x = belt2_center_x;
    target_y = belt2_end_y + side_y * (belt2_entry_gap + slot_pitch * (k - 1) + moving_stop_margin);
end

% Segment 1: Belt4
if s <= seg1_end
    ratio = safeRatio(s, seg1_end);

    x = belt4_center_x;
    y = belt4_start_y + ratio * (belt4_end_y - belt4_start_y);

    % Belt4: 짧은 변이 y방향
    yaw_rad = pi/2;

% Segment 2: Belt1
elseif s <= seg2_end
    local_s = s - seg1_end;
    seg_len = seg2_end - seg1_end;
    ratio = safeRatio(local_s, seg_len);

    x = belt1_right_x - ratio * (belt1_right_x - belt1_left_x);
    y = belt1_center_y;

    % Belt1: 짧은 변이 x방향
    yaw_rad = 0;

% Segment 3: Belt2 또는 Belt2 일부
elseif s <= seg3_end
    local_s = s - seg2_end;
    seg_len = seg3_end - seg2_end;
    ratio = safeRatio(local_s, seg_len);

    if target_slot <= max_on_belt3
        % Belt2 전체 이동
        x = belt2_center_x;
        y = belt2_start_y + ratio * (belt2_end_y - belt2_start_y);
    else
        % Belt2 위 목표 위치까지만 이동
        x = belt2_center_x;
        y = belt2_start_y + ratio * (target_y - belt2_start_y);
    end

    % Belt2: 짧은 변이 y방향
    yaw_rad = pi/2;

% Segment 4: Belt3
else
    local_s = s - seg3_end;

    % Belt3 진입점은 belt3_left_x, 목표는 target_x
    seg_len = abs(target_x - belt3_left_x);
    ratio = safeRatio(local_s, seg_len);

    x = belt3_left_x + ratio * (target_x - belt3_left_x);
    y = belt3_center_y;

    % Belt3: 짧은 변이 x방향
    yaw_rad = 0;
end

end


function r = safeRatio(a, b)
% 0~1 비율 계산

if b <= 0
    r = 1;
else
    r = a / b;
end

if r < 0
    r = 0;
end

if r > 1
    r = 1;
end

end

function a = wrapToPiLocal(a)
% wrapToPiLocal
% angle을 -pi ~ pi 범위로 정규화

while a > pi
    a = a - 2*pi;
end

while a < -pi
    a = a + 2*pi;
end

end

== matlab function baseline_auto_parcel_loading_process/Floor3VisualStateFunction ==
  data: floor3_queue input; floor3_visual_id output size=[6 1]; visual_shift_f3 input; target_id_f3 input; target_on_belt4_f3 input; current_unload_id input; package_on_platform_from_floor input; unload_done input; floor3_visual_path output size=[6 1]; floor3_visual_count output size=[1 1]; belt4_reverse_cmd input; belt4_restore_cmd input; belt4_reverse_progress output size=[1 1]; belt4_reverse_phase output size=[1 1]
function [floor3_visual_id, floor3_visual_path, floor3_visual_count, belt4_reverse_progress, belt4_reverse_phase] = ...
    Floor3VisualStateFunction(floor3_queue, visual_shift_f3, target_id_f3, target_on_belt4_f3, ...
                              current_unload_id, package_on_platform_from_floor, unload_done, ...
                              belt4_reverse_cmd, belt4_restore_cmd)
% Floor3VisualStateFunction
%
% 목적:
% - 3층 박스들의 시각적 벨트 위치를 따로 저장한다.
% - floor3_queue는 논리 queue이므로 하차 완료 시 압축될 수 있다.
% - visual state는 실제 벨트 위 위치를 유지한다.
%
% 핵심:
% - queue에 없다는 이유로 visual state에서 제거하지 않는다.
% - 실제 하차 완료된 carried_id만 unload_done 상승엣지에서 삭제한다.
% - Belt4 reverse/restore는 3층 하차 대상일 때만 동작한다.
% - reverse_progress는 persistent로 유지되어야 하며 매 스텝 초기화하면 안 된다.

MAX_VISUAL = 6;
QUEUE_MAX = 50;

persistent ids
persistent paths
persistent prev_shift
persistent initialized
persistent carried_id
persistent prev_unload_done

persistent reverse_progress
persistent reverse_phase
persistent prev_reverse_cmd
persistent prev_restore_cmd

if isempty(initialized)
    ids = zeros(MAX_VISUAL, 1);
    paths = zeros(MAX_VISUAL, 1);
    prev_shift = 0;
    initialized = 1;

    carried_id = 0;
    prev_unload_done = 0;

    reverse_progress = 0;
    reverse_phase = 0;
    prev_reverse_cmd = 0;
    prev_restore_cmd = 0;
end

% =========================
% 기본 출력 초기화
% =========================
floor3_visual_id = zeros(MAX_VISUAL, 1);
floor3_visual_path = zeros(MAX_VISUAL, 1);
floor3_visual_count = 0;

belt4_reverse_progress = reverse_progress;
belt4_reverse_phase = reverse_phase;

% =========================
% 1. queue에 새로 생긴 package를 visual state에 등록
% =========================
for q = 1:QUEUE_MAX
    pkg_id = floor3_queue(q);

    if pkg_id > 0
        exists = 0;

        for k = 1:MAX_VISUAL
            if ids(k) == pkg_id
                exists = 1;
            end
        end

        if exists < 0.5
            free_idx = 0;

            for k = 1:MAX_VISUAL
                if ids(k) <= 0 && free_idx == 0
                    free_idx = k;
                end
            end

            if free_idx > 0
                ids(free_idx) = pkg_id;
                paths(free_idx) = q;
            end
        end
    end
end

% =========================
% 2. queue에서 사라진 package 제거 금지
% =========================
% floor3_queue는 논리 queue이므로 하차 완료 후 압축될 수 있다.
% visual state는 실제 벨트 위 위치를 표현하므로,
% queue에 없다는 이유만으로 삭제하지 않는다.

% =========================
% 3. 플랫폼 위에 올라간 package ID 기억
% =========================
if package_on_platform_from_floor > 0.5 && current_unload_id > 0
    carried_id = current_unload_id;
end

% =========================
% 4. unload_done 상승엣지에서 carried_id 제거
% =========================
unload_done_rise = 0;

if unload_done > 0.5 && prev_unload_done <= 0.5
    unload_done_rise = 1;
end

if unload_done_rise > 0.5 && carried_id > 0
    for k = 1:MAX_VISUAL
        if ids(k) == carried_id
            ids(k) = 0;
            paths(k) = 0;
        end
    end

    carried_id = 0;
end

prev_unload_done = unload_done;

% =========================
% 5. visual_shift 변화량으로 모든 박스 이동
% =========================
delta = visual_shift_f3 - prev_shift;

% target 전환 시 visual_shift가 리셋되면 뒤로 돌아가지 않게 한다.
if delta < 0
    delta = 0;
    prev_shift = visual_shift_f3;
end

% 너무 큰 점프 방지
if delta > 1
    delta = 1;
end

% target이 하차공간을 지나 과도하게 이동하지 않도록 제한
if delta > 0
    target_path = 999;

    if target_id_f3 > 0
        for k = 1:MAX_VISUAL
            if ids(k) == target_id_f3
                target_path = paths(k);
            end
        end
    end

    if target_path <= 0
        delta = 0;
    elseif delta > target_path
        delta = target_path;
    end
end

% 준비 완료 상태에서는 더 이상 하차공간 방향 순환 이동을 하지 않음
if target_on_belt4_f3 > 0.5
    delta = 0;
end

if delta > 0
    for k = 1:MAX_VISUAL
        if ids(k) > 0
            paths(k) = paths(k) - delta;
        end
    end
end

if visual_shift_f3 >= prev_shift
    prev_shift = visual_shift_f3;
end

% =========================
% 6. Belt4 reverse/restore 동작
% =========================
% reverse_progress = 0 : Belt4 원위치
% reverse_progress = 1 : 하차 대상 박스가 플랫폼 위로 충분히 밀린 상태
%
% 중요:
% - belt4_reverse_cmd는 전 층 공통 신호일 수 있으므로,
%   3층 하차 대상일 때만 local_reverse_cmd를 허용한다.
% - restore는 reverse_progress가 실제로 0보다 클 때만 허용한다.
% - reverse_cmd가 짧게 들어와도 reverse_phase가 latch되어 1까지 진행된다.

Ts_reverse = 0.05;
reverse_speed = 0.30;
reverse_step = reverse_speed * Ts_reverse;

is_current_floor3_unload = 0;

if target_id_f3 > 0 && current_unload_id > 0
    if target_id_f3 == current_unload_id
        is_current_floor3_unload = 1;
    end
end

local_reverse_cmd = 0;
local_restore_cmd = 0;

% 3층 대상이 하차공간에 있고, 현재 하차 대상도 3층 target일 때만 reverse 시작
if belt4_reverse_cmd > 0.5 && is_current_floor3_unload > 0.5 && target_on_belt4_f3 > 0.5
    local_reverse_cmd = 1;
end

% reverse_progress가 실제로 진행된 층만 restore 허용
if belt4_restore_cmd > 0.5 && reverse_progress > 0
    local_restore_cmd = 1;
end

reverse_cmd_rise = 0;
restore_cmd_rise = 0;

if local_reverse_cmd > 0.5 && prev_reverse_cmd <= 0.5
    reverse_cmd_rise = 1;
end

if local_restore_cmd > 0.5 && prev_restore_cmd <= 0.5
    restore_cmd_rise = 1;
end

prev_reverse_cmd = local_reverse_cmd;
prev_restore_cmd = local_restore_cmd;

if reverse_cmd_rise > 0.5
    reverse_phase = 1;
end

if restore_cmd_rise > 0.5
    reverse_phase = 2;
end

if reverse_phase == 1

    reverse_progress = reverse_progress + reverse_step;

    if reverse_progress >= 1
        reverse_progress = 1;
        reverse_phase = 0;
    end

elseif reverse_phase == 2

    reverse_progress = reverse_progress - reverse_step;

    if reverse_progress <= 0
        reverse_progress = 0;
        reverse_phase = 0;
    end

end

belt4_reverse_progress = reverse_progress;
belt4_reverse_phase = reverse_phase;

% =========================
% 7. 출력 정리
% =========================
count = 0;

% 하차 대상이 아닌 Belt4 위 박스들의 역회전 표시 이동량
% 너무 크게 주면 path가 0을 넘어 Belt3 위치로 넘어가 보인다.
NON_TARGET_REVERSE_TRAVEL = 1.5;

for k = 1:MAX_VISUAL
    floor3_visual_id(k) = ids(k);

    display_path = paths(k);

    if reverse_progress > 0
        if ids(k) > 0 && paths(k) <= 0

            % 현재 하차 대상은 F3 makePkg에서 handoff -> platform으로 별도 표시한다.
            % 여기서는 하차 대상이 아닌 Belt4 위 박스만 살짝 밀었다가 복귀시킨다.
            if ids(k) ~= current_unload_id
                display_path = paths(k) + reverse_progress * NON_TARGET_REVERSE_TRAVEL;

                % path > 0이 되면 Belt3 슬롯으로 해석되므로 방지한다.
                if display_path > -0.05
                    display_path = -0.05;
                end
            end
        end
    end

    floor3_visual_path(k) = display_path;

    if ids(k) > 0
        count = count + 1;
    end
end

floor3_visual_count = count;

end
